simulink model "CasterFSMStandalone"  (Simulink 8.0)
settings: Solver=ode3  StartTime=0.0  StopTime=inf  FixedStep=0.001  RelTol=1e-3
undefined symbols (not defined in the file): load_caster_fsm_settings
settings Model: Creator=caster  LastModifiedBy=caster

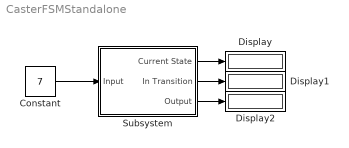
== system CasterFSMStandalone ==
  Constant : Constant  Value=7
  Display : Display
  Display1 : Display
  Display2 : Display
  Subsystem : Subsystem
  wires:
  Constant/1 -> Subsystem/1(Input)
  Subsystem/1(Current State) -> Display/1
  Subsystem/2(In Transition) -> Display1/1
  Subsystem/3(Output) -> Display2/1

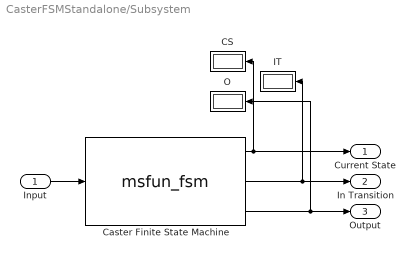
== system CasterFSMStandalone/Subsystem ==
  Input : Inport
  CS : Display
  Caster Finite State Machine : M-S-Function  FunctionName=msfun_fsm  Parameters=nsts, outs, initState, ansts, irp, errortrans  mask(Finite State Machine){initState=load_caster_fsm_settings('Initial State');, outs=load_caster_fsm_settings('Output Functions');, nsts=load_caster_fsm_settings('Next State Transitions');, errortrans=load_caster_fsm_settings('Error Transitions');, ansts=load_caster_fsm_settings('Absolute Next State Transitions');, irp=on}
      mask prompts: initState "Initial State:"; outs "Output Functions"; nsts "Next State Transitions"; errortrans "Error Transitions"; ansts "Absolute Next-State Transitions"; irp "Ignore Repeated Inputs?"
      mask help: This block allows one to enter in various parameters of a finite state machine.
      mask Display:
      | port_label('input',1,'Input Signals');
      | port_label('output',1,'Current State');
      | port_label('output',2,'In-transition');
      | port_label('output',3,'Output Signal');
  IT : Display
  O : Display
  Current State : Outport
  In Transition : Outport  Port=2
  Output : Outport  Port=3
  wires:
  Input/1 -> Caster Finite State Machine/1
  Caster Finite State Machine/1 -> Current State/1, CS/1
  Caster Finite State Machine/2 -> In Transition/1, IT/1
  Caster Finite State Machine/3 -> Output/1, O/1
